simulink model "eFL_regulacija_nelin_sim"  (R2020a)
settings: Solver=ode5  StartTime=0.0  StopTime=tfin  FixedStep=1e-4  RelTol=1e-3
values from neighbouring files (symbols this model uses):
  disturb_S = 0    [eFL_regulacija_nelin_sim_matlab.m]    (also in robusna_of_eFL_regulacija_nelin_sim_matlab.m)
  disturb_X = 0.2*Xe    (= 0.97814)    [eFL_regulacija_nelin_sim_matlab.m]    (also in robusna_of_eFL_regulacija_nelin_sim_matlab.m = 0)
  F_lower_limit = 0    [eFL_regulacija_nelin_sim_matlab.m]    (also in robusna_of_eFL_regulacija_nelin_sim_matlab.m)
  F_upper_limit = Fe+1e-3*Fe    (= 3.2121089)    [eFL_regulacija_nelin_sim_matlab.m]    (also in robusna_of_eFL_regulacija_nelin_sim_matlab.m)
  K0_FLIRT = 2.2548    [eFL_regulacija_nelin_sim_matlab.m]    (also in robusna_of_eFL_regulacija_nelin_sim_matlab.m)
  K0_FLRT = w0    (= 0.5637)    [eFL_regulacija_nelin_sim_matlab.m]    (also in robusna_of_eFL_regulacija_nelin_sim_matlab.m)
  K1 = 0.03    [eFL_regulacija_nelin_sim_matlab.m]    (also in robusna_of_eFL_regulacija_nelin_sim_matlab.m)
  K2 = 0.5    [eFL_regulacija_nelin_sim_matlab.m]    (also in robusna_of_eFL_regulacija_nelin_sim_matlab.m)
  Ki = 1.27    [eFL_regulacija_nelin_sim_matlab.m]    (also in robusna_of_eFL_regulacija_nelin_sim_matlab.m)
  mi_max = 1    [eFL_regulacija_nelin_sim_matlab.m]    (also in robusna_of_eFL_regulacija_nelin_sim_matlab.m)
  S_step = 0    [eFL_regulacija_nelin_sim_matlab.m]    (also in robusna_of_eFL_regulacija_nelin_sim_matlab.m = 0.0138)
  S_time_step1 = 2    [eFL_regulacija_nelin_sim_matlab.m]    (also in robusna_of_eFL_regulacija_nelin_sim_matlab.m = 20)
  S_time_step2 = 40    [eFL_regulacija_nelin_sim_matlab.m]    (also in robusna_of_eFL_regulacija_nelin_sim_matlab.m = 50)
  Se = 0.2187    [eFL_regulacija_nelin_sim_matlab.m]    (also in robusna_of_eFL_regulacija_nelin_sim_matlab.m)
  SF = 10    [eFL_regulacija_nelin_sim_matlab.m]    (also in robusna_of_eFL_regulacija_nelin_sim_matlab.m)
  std_noise = 1e-5*Se    (= 2.187e-06)    [eFL_regulacija_nelin_sim_matlab.m]    (also in robusna_of_eFL_regulacija_nelin_sim_matlab.m = 0)
  V = 4    [eFL_regulacija_nelin_sim_matlab.m]    (also in robusna_of_eFL_regulacija_nelin_sim_matlab.m)
  x10 = Xe    (= 4.8907)    [eFL_regulacija_nelin_sim_matlab.m]    (also in robusna_of_eFL_regulacija_nelin_sim_matlab.m)
  x20 = Se    (= 0.2187)    [eFL_regulacija_nelin_sim_matlab.m]    (also in robusna_of_eFL_regulacija_nelin_sim_matlab.m)
  Y = 0.5    [eFL_regulacija_nelin_sim_matlab.m]    (also in robusna_of_eFL_regulacija_nelin_sim_matlab.m)
undefined symbols (not defined in the file or in its folder): magnitude
settings Model: Creator=anaMceranic  LastModifiedBy=anaMceranic
settings DataIOCC: ReturnWorkspaceOutputs=off

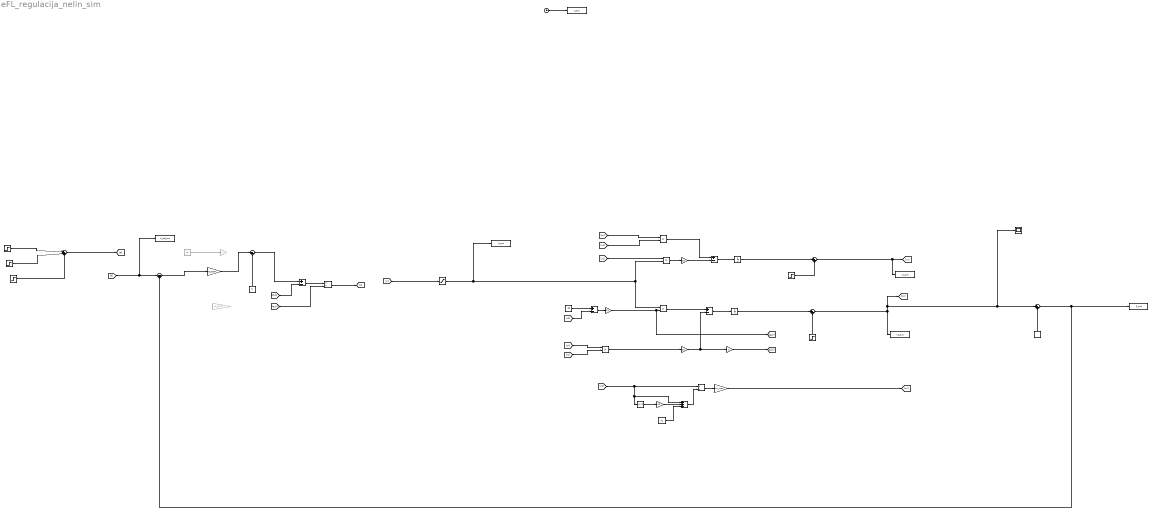
== system eFL_regulacija_nelin_sim ==
  note: eFL
  note: Subsystem1
  note: eFL
  Add : Sum  Inputs=+-
  Add1 : Sum  Inputs=+-
  Add2 : Sum  Inputs=+++
  Add3 : Sum  Inputs=+-
  Clock : Clock
  Constant : Constant  Value=K1
  Constant1 : Constant  Value=0
  Constant2 : Constant  Value=SF
  Divide : Product  Inputs=*/
  Divide1 : Product  Inputs=*/
  Gain : Gain  Commented=on  Gain=K0_FLIRT
  Gain1 : Gain  Gain=-1
  Gain2 : Gain  Commented=on  Gain=Ki
  Gain3 : Gain  Gain=K0_FLRT
  Integrator : Integrator  InitialCondition=x10
  Integrator1 : Integrator  InitialCondition=x20
  Integrator2 : Integrator  Commented=on
  Multiply : Gain  Gain=1/V
  Multiply2 : Gain  Gain=1/Y
  Multiply3 : Gain  Gain=mi_max
  Multiply4 : Gain  Gain=K2
  Multiply6 : Gain  Gain=1/V
  Power : Math  Operator=magnitude^2  SaturateOnIntegerOverflow=on
  Product{,1..3} (4 alike) : Product
  Random Number : RandomNumber  Variance=std_noise  SampleTime=0.1
  Saturation : Saturate  UpperLimit=F_upper_limit  LowerLimit=F_lower_limit
  Scope : Scope
  Step : Step  Time=5  After=disturb_X  SampleTime=0
  Step2 : Step  Time=0  Before=Se  After=Se  SampleTime=0
  Step3 : Step  Time=S_time_step1  After=S_step  SampleTime=0
  Step4 : Step  Time=S_time_step2  After=-S_step  SampleTime=0
  Step5 : Step  Time=5  After=disturb_S  SampleTime=0
  Subtract : Sum  Inputs=+-
  Sum : Sum  Inputs=|++
  Sum1 : Sum  Inputs=|--
  Sum2 : Sum  Inputs=|-+
  Sum3 : Sum  Inputs=|++
  Sum4 : Sum  Inputs=|++
  Sum7 : Sum  Inputs=|+++
  To Workspace : ToWorkspace  VariableName=x1_out  SampleTime=-1
  To Workspace1 : ToWorkspace  VariableName=t_out  SampleTime=-1
  To Workspace2 : ToWorkspace  VariableName=x2_out  SampleTime=-1
  To Workspace3 : ToWorkspace  VariableName=S_out  SampleTime=-1
  To Workspace4 : ToWorkspace  VariableName=S_ref_out  SampleTime=-1
  To Workspace7 : ToWorkspace  VariableName=F_out  SampleTime=-1
  wires:
  Clock/1 -> To Workspace1/1
  Sum7/1 -> [R]
  Step2/1 -> Sum7/1
  Step3/1 -> Sum7/2
  Step4/1 -> Sum7/3
  [x1] -> Product2/2
  Product2/1 -> Multiply2/1
  Multiply/1 -> Add/2
  Add2/1 -> Divide/2
  Constant/1 -> Add2/3
  [x1] -> Product3/2
  Multiply4/1 -> Add2/2
  [mi] -> Product2/1
  Multiply3/1 -> [mi]
  Power/1 -> Multiply4/1
  Constant2/1 -> Subtract/1
  [x2] -> Subtract/2
  Add1/1 -> Integrator1/1
  Multiply2/1 -> Gain1/1, Add1/2
  Divide/1 -> Multiply3/1
  Product3/1 -> Add/1
  [x1] -> Product/1
  Product1/1 -> Add1/1
  [x2] -> Power/1, Add2/1, Divide/1
  Add/1 -> Integrator/1
  Product/1 -> Multiply/1
  [mi] -> Product3/1
  Integrator/1 -> Sum/1
  Sum/1 -> [x1], To Workspace/1
  Step/1 -> Sum/2
  Gain1/1 -> [Lf_h]
  Subtract/1 -> Multiply6/1
  Multiply6/1 -> [Lg_h], Product1/2
  [Lf_h] -> Add3/2
  Add3/1 -> Divide1/1
  [Lg_h] -> Divide1/2
  Divide1/1 -> [u]
  [R] -> To Workspace4/1, Sum2/1
  Sum1/1 -> Add3/1
  Sum3/1 -> Sum2/2, To Workspace3/1
  Random Number/1 -> Sum3/2
  Step5/1 -> Sum4/2
  Integrator1/1 -> Sum4/1
  Sum4/1 -> Scope/1, Sum3/1, [x2], To Workspace2/1
  [u] -> Saturation/1
  Saturation/1 -> To Workspace7/1, Product1/1, Product/2
  Integrator2/1 -> Gain2/1
  Gain3/1 -> Sum1/1
  Sum2/1 -> Gain3/1
  Constant1/1 -> Sum1/2
